simulink model "FSK"  (R2024a)
settings: Solver=VariableStepAuto  StartTime=0.0  StopTime=10.0  RelTol=1e-3
settings Model: Creator=prath  LastModifiedBy=prath

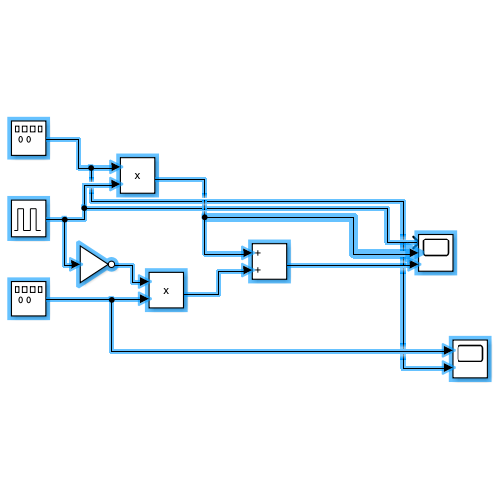
[thumbnail: Simulink's stored preview of the top-level diagram]
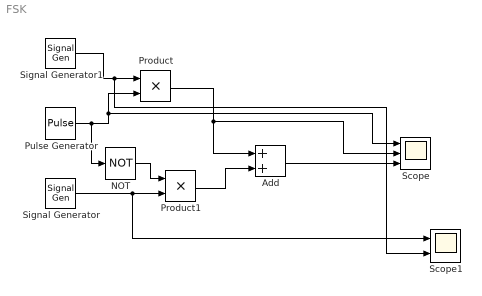
== system FSK ==
  Add : Sum
  NOT : Logic  Operator=NOT  IconShape=distinctive  AllPortsSameDT=off  OutDataTypeStr=boolean
  Product : Product
  Product1 : Product
  Pulse Generator : DiscretePulseGenerator  PulseType=Time based  PulseWidth=50
  Scope : Scope  NumInputPorts=3
  Scope1 : Scope  NumInputPorts=2
  Signal Generator : SignalGenerator  Frequency=5
  Signal Generator1 : SignalGenerator  Frequency=10  VectorParams1D=off
  wires:
  Add/1 -> Scope/3
  Signal Generator/1 -> Scope1/1, Product1/2
  Signal Generator1/1 -> Scope1/2, Product/1
  NOT/1 -> Product1/1
  Product1/1 -> Add/2
  Pulse Generator/1 -> NOT/1, Scope/1, Product/2
  Product/1 -> Scope/2, Add/1
